simulink library "wlan80211g_lib"  (Simulink 7.5)
settings: Solver=ode45  SolverMode=SingleTasking  StartTime=0.0  StopTime=10.0  RelTol=1e-3
libraries: commblkintrlv2 x4, commdigbbndam3 x3, commcnvcod2 x2, commutil2 x1, dspsigops x1
Description:
  | Library blocks for IEEE 802.11a model
settings Model: Creator=The MathWorks Inc.  LastModifiedBy=User  ExtModeAutoUpdateStatusClock=off

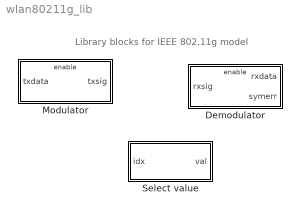
== system wlan80211g_lib ==
  note: Library blocks for IEEE 802.11g model
  Demodulator : Subsystem  mask(QAM Demodulator-Decoder.){numSymbols=960, modulation=OQPSK, code=3/4, trellisStructure=poly2trellis(7, [171 133]), punctureVector=[1 1 1 0 0 1].', vtbd=34}
      mask prompts: numSymbols "Number of symbols per frame:"; trellisStructure "Trellis:"; punctureVector "Puncture vector:"; vtbd "Viterbi trace back depth:"
      mask help: Demodulator has option to zero-pad output, so that a bank of different modulators can share the same output frame size.
      mask init:
      | % number of bits per symbol
      | switch modulation
      | 	case 'BPSK', Nb1 = 1;
      | 	case 'QPSK', Nb1 = 2;
      | 	case '16-QAM', Nb1 = 4;
      | 	case '64-QAM', Nb1 = 6;
      |     case 'DQPSK', Nb1 = 8;
      |     case 'OQPSK', Nb1 = 16;
      | end
      | 
      | modOrder = 2.^Nb1;
      | Nb = numSymbols * Nb1; % tx bits per block
      | codeRate = str2num(strvcat(code)).';
      | bitsPerBlock = Nb .* codeRate;
      | 
      | % interleaver
      | interleaverRows = 16;
      | if rem(Nb, interleaverRows)
      | 	error('commblks:commwlan80211a_lib:InvalidNumTxBits',...
      |           'Number of transmitted bits per block must be multiple of 16.')
      | end
      | interleaverCols = Nb / interleaverRows;
      | interleaverElements = [...
      |             2*floor( [0:Nb-1]/2 ) + ...
      |             mod( ([0:Nb-1] + Nb - floor( interleaverRows*[0:Nb-1]/Nb ) ), 2 ) ...
      |             + 1]';
      mask Display:
      | disp(['Demodulator\n' modulation ' ' code])
      | port_label('input', 1, ' ')
      | port_label('output', 1, ' ')
      | port_label('output', 2, 'err')
  Modulator : Subsystem  mask(Modulator-Coder.){numSymbols=960, modulation=OQPSK, code=3/4, trellisStructure=poly2trellis(7, [171 133]), punctureVector=[1 1 1 0 0 1].'}
      mask prompts: numSymbols "Number of symbols per frame:"; trellisStructure "Trellis:"; punctureVector "Puncture vector:"
      mask help: Modulator gates incoming bits so that a bank of different modulators can share the same input frame size.
      mask init:
      | % number of bits per symbol
      | switch modulation
      | 	case 'BPSK', Nb1 = 1;
      | 	case 'QPSK', Nb1 = 2;
      | 	case '16-QAM', Nb1 = 4;
      | 	case '64-QAM', Nb1 = 6;
      |     case 'DQPSK', Nb1 = 8;
      |     case 'OQPSK', Nb1 = 16;
      |         
      | end
      | 
      | modOrder = 2.^Nb1;
      | Nb = numSymbols * Nb1; % tx bits per block
      | codeRate = str2num(strvcat(code)).';
      | bitsPerBlock = Nb .* codeRate;
      | 
      | % interleaver
      | interleaverRows = 16;
      | if rem(Nb, interleaverRows)
      | 	error('commblks:commwlan80211a_lib:InvalidNumTxBits',...
      |           'Number of transmitted bits per block must be multiple of 16.')
      | end
      | interleaverCols = Nb / interleaverRows;
      | interleaverElements = [...
      |             2*floor( [0:Nb-1]/2 ) + ...
      |             mod( ([0:Nb-1] + Nb - floor( interleaverRows*[0:Nb-1]/Nb ) ), 2 ) ...
      |             + 1]';
      mask Display: disp(['Modulator\n' modulation ' ' code])
  Select value : Subsystem  mask{vector=[0 1 2 3]}
      mask help: Using MATLAB-style indexing, output value of selected element of vector.
      mask Display: disp('Select\nValue')

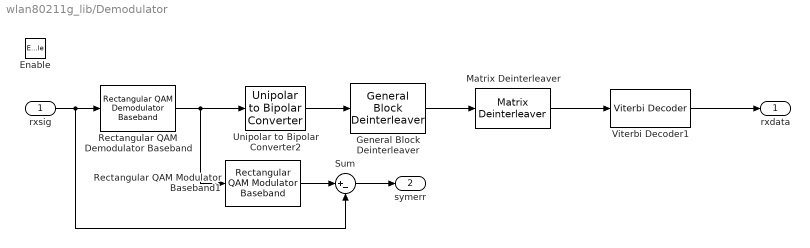
== system wlan80211g_lib/Demodulator ==
  rxsig : Inport  OutDataType=sfix(16)  OutScaling=2^0
  Enable : EnablePort
  General Block Deinterleaver : commblkintrlv2/General Block Deinterleaver  elements=interleaverElements
  Matrix Deinterleaver : commblkintrlv2/Matrix Deinterleaver  SystemSampleTime=-1  Nrows=interleaverRows  Ncols=interleaverCols
  Rectangular QAM Demodulator Baseband : commdigbbndam3/Rectangular QAM Demodulator Baseband  DialogController=commDDGCreate  DialogControllerArgs=DataTag0  M=modOrder  PowType=Average Power  MinDist=2  AvgPow=1  PeakPow=1  Ph=0  Dec=Gray  Mapping=[0:15]  OutType=Bit  DecType=Hard decision  VarSource=Dialog  Variance=1  outDtype1=double  outDtype2=double  derotateFactorWordLen=16  denormFactorWordLen=16  prodOutWordLen=32  prodOutRoundingMode=Floor  prodOutOverflowMode=Wrap  sumWordLen=32
  Rectangular QAM Modulator Baseband1 : commdigbbndam3/Rectangular QAM Modulator Baseband  DialogController=commDDGCreate  DialogControllerArgs=DataTag1  M=modOrder  InType=Bit  Enc=Gray  Mapping=[0:15]  PowType=Average Power  MinDist=2  AvgPow=1  PeakPow=1  Ph=0  outDtype=double  outWordLen=16  outUDDataType=sfix(16)  outFracLenMode=Best precision  outFracLen=15
  Sum : Sum  Inputs=|+-  OutDataType=sfix(16)  OutScaling=2^0  SaturateOnIntegerOverflow=on
  Unipolar to Bipolar Converter2 : commutil2/Unipolar to Bipolar Converter  SystemSampleTime=-1  M=2  polarity=Negative  dataType=Inherit via internal rule
  Viterbi Decoder1 : commcnvcod2/Viterbi Decoder  DialogController=commDDGCreate  DialogControllerArgs=DataTag2  trellis=trellisStructure  isPunctured=on  punctureVector=punctureVector  erasures=off  dectype=Unquantized  runSigValErrCheck=off  nsdecb=4  smWordLength=16  tbdepth=vtbd  opmode=Continuous  reset=off  outDataType=double
  rxdata : Outport  OutDataType=sfix(16)  OutScaling=2^0  OutputWhenDisabled=reset  InitialOutput=0
  symerr : Outport  Port=2  OutDataType=sfix(16)  OutScaling=2^0  OutputWhenDisabled=reset  InitialOutput=0
  wires:
  Rectangular QAM Demodulator Baseband/1 -> Unipolar to Bipolar Converter2/1, Rectangular QAM Modulator Baseband1/1
  rxsig/1 -> Rectangular QAM Demodulator Baseband/1, Sum/2
  Unipolar to Bipolar Converter2/1 -> General Block Deinterleaver/1
  Viterbi Decoder1/1 -> rxdata/1
  Rectangular QAM Modulator Baseband1/1 -> Sum/1
  Sum/1 -> symerr/1
  Matrix Deinterleaver/1 -> Viterbi Decoder1/1
  General Block Deinterleaver/1 -> Matrix Deinterleaver/1

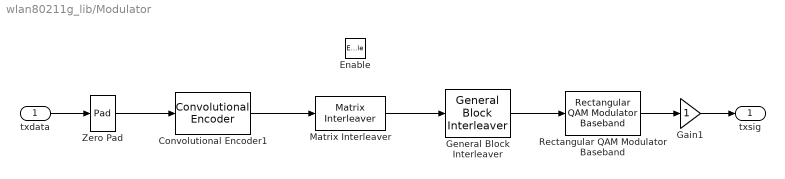
== system wlan80211g_lib/Modulator ==
  txdata : Inport  OutDataType=sfix(16)  OutScaling=2^0
  Enable : EnablePort
  Convolutional Encoder1 : commcnvcod2/Convolutional Encoder  trellis=trellisStructure  opMode=Continuous  hasIniStPort=off  hasFinStPort=off  usePuncVector=on  punctureVector=punctureVector  reset=Unused parameter value
  Gain1 : Gain  ParameterDataType=sfix(16)  ParameterScaling=2^0  OutDataType=sfix(16)  OutScaling=2^0  SaturateOnIntegerOverflow=on  OutDataTypeStr=Inherit: Same as input  ParamDataTypeStr=Inherit: Same as input
  General Block Interleaver : commblkintrlv2/General Block Interleaver  elements=interleaverElements
  Matrix Interleaver : commblkintrlv2/Matrix Interleaver  SystemSampleTime=-1  Nrows=interleaverRows  Ncols=interleaverCols
  Rectangular QAM Modulator Baseband : commdigbbndam3/Rectangular QAM Modulator Baseband  DialogController=commDDGCreate  DialogControllerArgs=DataTag3  M=modOrder  InType=Bit  Enc=Gray  Mapping=[0:15]  PowType=Average Power  MinDist=2  AvgPow=1  PeakPow=1  Ph=0  outDtype=double  outWordLen=16  outUDDataType=sfix(16)  outFracLenMode=Best precision  outFracLen=15
  Zero Pad : dspsigops/Pad  padAlong=Columns  dimsToPad=1  valSrc=Specify via dialog  padVal=0  spec=Output size  padNumOutRowsSpecMethod=User-specified  numOutRows=bitsPerBlock  padNumOutColsSpecMethod=User-specified  numOutCols=1  isVarDimsMode=off  padBeginning=0  padEnd=0  outSizeMode=User-specified  outSize=1  padSigAt=End  trunc_flag=None  roundingMode=Floor  overflowMode=off  truncOrWrapMode=Truncate  wrap_flag=None
      settings: AttributesFormatString=\n
  txsig : Outport  OutDataType=sfix(16)  OutScaling=2^0
  wires:
  General Block Interleaver/1 -> Rectangular QAM Modulator Baseband/1
  Matrix Interleaver/1 -> General Block Interleaver/1
  Convolutional Encoder1/1 -> Matrix Interleaver/1
  Zero Pad/1 -> Convolutional Encoder1/1
  txdata/1 -> Zero Pad/1
  Gain1/1 -> txsig/1
  Rectangular QAM Modulator Baseband/1 -> Gain1/1

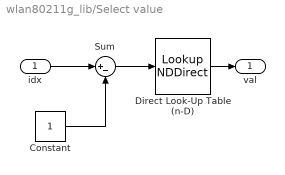
== system wlan80211g_lib/Select value ==
  idx : Inport  OutDataType=sfix(16)  OutScaling=2^0
  Constant : Constant  OutDataType=sfix(16)  OutScaling=2^0
  Direct Look-Up Table (n-D) : LookupNDDirect  NumberOfTableDimensions=1  Table=vector
  Sum : Sum  Inputs=|+-  OutDataType=sfix(16)  OutScaling=2^0  SaturateOnIntegerOverflow=on
  val : Outport  OutDataType=sfix(16)  OutScaling=2^0
  wires:
  Constant/1 -> Sum/2
  Sum/1 -> Direct Look-Up Table (n-D)/1
  Direct Look-Up Table (n-D)/1 -> val/1
  idx/1 -> Sum/1
